simulink model "frequency_synth"  (R2020a)
settings: Solver=VariableStepAuto  StartTime=0.0  StopTime=inf  RelTol=1e-3
undefined symbols (not defined in the file): df
libraries: hdlsllib x36, dsphdlsigops x4
settings Model: Creator=david  LastModifiedBy=david
settings OptimizationCC: BlockReduction=off  ConditionallyExecuteInputs=off  DefaultParameterBehavior=Inlined
settings DebuggingCC: AlgebraicLoopMsg=error
settings HardwareCC: ProdBitPerPointer=32  ProdBitPerSizeT=32  ProdBitPerPtrDiffT=32  ProdLargestAtomicFloat=None  ProdIntDivRoundTo=Undefined  ProdEndianess=Unspecified  ProdWordSize=32  ProdHWDeviceType=ASIC/FPGA->ASIC/FPGA  TargetBitPerPointer=64  TargetBitPerSizeT=64  TargetBitPerPtrDiffT=64  TargetLongLongMode=on  TargetIntDivRoundTo=Zero  TargetEndianess=LittleEndian  TargetWordSize=64  TargetHWDeviceType=Custom Processor->MATLAB Host Computer  ProdEqTarget=off

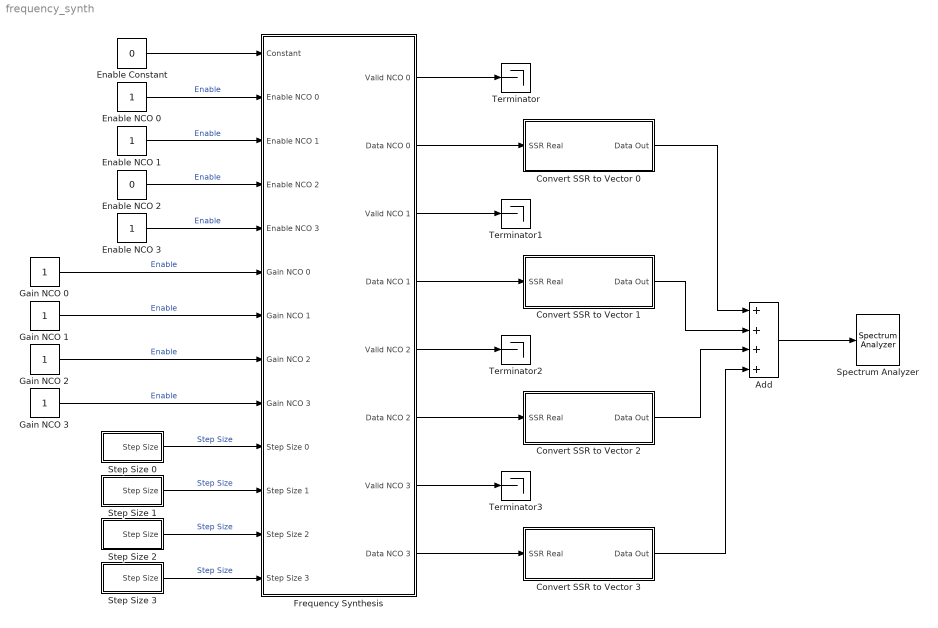
== system frequency_synth ==
  Add : Sum  Inputs=++++
  Convert SSR to Vector 0 : Subsystem
  Convert SSR to Vector 1 : Subsystem
  Convert SSR to Vector 2 : Subsystem
  Convert SSR to Vector 3 : Subsystem
  Enable Constant : Constant  Value=0  OutDataTypeStr=uint32  SampleTime=-1
  Enable NCO 0 : Constant  OutDataTypeStr=boolean  SampleTime=-1
  Enable NCO 1 : Constant  OutDataTypeStr=boolean  SampleTime=-1
  Enable NCO 2 : Constant  Value=0  OutDataTypeStr=boolean  SampleTime=-1
  Enable NCO 3 : Constant  OutDataTypeStr=boolean  SampleTime=-1
  Frequency Synthesis : Subsystem  TreatAsAtomicUnit=on
  Gain NCO {0..3} (4 alike) : Constant  OutDataTypeStr=fixdt(1,16,14)  SampleTime=-1
  Spectrum Analyzer : SpectrumAnalyzer
  Step Size 0 : Subsystem  mask{fs=1.024e9, f=20.1e6, b=32, i=16, ssr=4}
      mask prompts: fs "Sample Frequency (Hz):"; f "Desired Frequency (Hz):"; b "Accumulator Bits:"; i "Quantized Bits:"; ssr "Sample per clock cycle:"
      mask init:
      | N = 2^i;
      | df = (f/fs)*N * 2^(b-i);
  Step Size 1 : Subsystem  mask{fs=1.024e9, f=40.1e6, b=32, i=16, ssr=4}
      mask prompts: fs "Sample Frequency (Hz):"; f "Desired Frequency (Hz):"; b "Accumulator Bits:"; i "Quantized Bits:"; ssr "Sample per clock cycle:"
      mask init:
      | N = 2^i;
      | df = (f/fs)*N * 2^(b-i);
  Step Size 2 : Subsystem  mask{fs=1.024e9, f=80.1e6, b=32, i=16, ssr=4}
      mask prompts: fs "Sample Frequency (Hz):"; f "Desired Frequency (Hz):"; b "Accumulator Bits:"; i "Quantized Bits:"; ssr "Sample per clock cycle:"
      mask init:
      | N = 2^i;
      | df = (f/fs)*N * 2^(b-i);
  Step Size 3 : Subsystem  mask{fs=1.024e9, f=450.01e6, b=32, i=16, ssr=4}
      mask prompts: fs "Sample Frequency (Hz):"; f "Desired Frequency (Hz):"; b "Accumulator Bits:"; i "Quantized Bits:"; ssr "Sample per clock cycle:"
      mask init:
      | N = 2^i;
      | df = (f/fs)*N * 2^(b-i);
  Terminator{,1..3} (4 alike) : Terminator
  wires:
  Step Size 0/1(Step Size) -> Frequency Synthesis/10(Step Size 0)  "Step Size"
  Enable NCO 0/1 -> Frequency Synthesis/2(Enable NCO 0)  "Enable"
  Step Size 1/1(Step Size) -> Frequency Synthesis/11(Step Size 1)  "Step Size"
  Frequency Synthesis/2(Data NCO 0) -> Convert SSR to Vector 0/1(SSR Real)
  Step Size 2/1(Step Size) -> Frequency Synthesis/12(Step Size 2)  "Step Size"
  Step Size 3/1(Step Size) -> Frequency Synthesis/13(Step Size 3)  "Step Size"
  Enable NCO 1/1 -> Frequency Synthesis/3(Enable NCO 1)  "Enable"
  Enable NCO 2/1 -> Frequency Synthesis/4(Enable NCO 2)  "Enable"
  Enable NCO 3/1 -> Frequency Synthesis/5(Enable NCO 3)  "Enable"
  Gain NCO 3/1 -> Frequency Synthesis/9(Gain NCO 3)  "Enable"
  Gain NCO 0/1 -> Frequency Synthesis/6(Gain NCO 0)  "Enable"
  Gain NCO 1/1 -> Frequency Synthesis/7(Gain NCO 1)  "Enable"
  Gain NCO 2/1 -> Frequency Synthesis/8(Gain NCO 2)  "Enable"
  Frequency Synthesis/1(Valid NCO 0) -> Terminator/1
  Frequency Synthesis/3(Valid NCO 1) -> Terminator1/1
  Frequency Synthesis/5(Valid NCO 2) -> Terminator2/1
  Frequency Synthesis/7(Valid NCO 3) -> Terminator3/1
  Add/1 -> Spectrum Analyzer/1
  Convert SSR to Vector 0/1(Data Out) -> Add/1
  Frequency Synthesis/4(Data NCO 1) -> Convert SSR to Vector 1/1(SSR Real)
  Convert SSR to Vector 1/1(Data Out) -> Add/2
  Frequency Synthesis/6(Data NCO 2) -> Convert SSR to Vector 2/1(SSR Real)
  Convert SSR to Vector 2/1(Data Out) -> Add/3
  Frequency Synthesis/8(Data NCO 3) -> Convert SSR to Vector 3/1(SSR Real)
  Convert SSR to Vector 3/1(Data Out) -> Add/4
  Enable Constant/1 -> Frequency Synthesis/1(Constant)

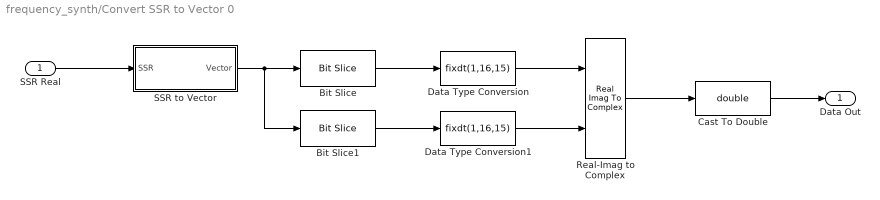
== system frequency_synth/Convert SSR to Vector 0 ==
  SSR Real : Inport
  Bit Slice : hdlsllib/Logic and Bit Operations/Bit Slice  lidx=15  ridx=0
      settings: SourceProductBaseCode=SL
  Bit Slice1 : hdlsllib/Logic and Bit Operations/Bit Slice  lidx=31  ridx=16
      settings: SourceProductBaseCode=SL
  Cast To Double : DataTypeConversion  OutDataTypeStr=double
  Data Type Conversion : DataTypeConversion  OutDataTypeStr=fixdt(1,16,15)  ConvertRealWorld=Stored Integer (SI)
  Data Type Conversion1 : DataTypeConversion  OutDataTypeStr=fixdt(1,16,15)  ConvertRealWorld=Stored Integer (SI)
  Real-Imag to Complex : RealImagToComplex
  SSR to Vector : Subsystem  mask{N=4, w=32, hN=4, hw=32}
      mask prompts: N "Samples per clock cycle:"; w "Wordlength:"
      mask init:
      | if ~isequal(get_param(gcb, 'N'), get_param(gcb, 'hN')) ||...
      |         ~isequal(get_param(gcb, 'w'), get_param(gcb, 'hw'))
      |     % Delete all blocks except input and output ports
      |     delete_block(setxor(setdiff(...
      |         find_system(gcb,'LookUnderMasks','on'),...
      |         {[gcb, '/Vector'], [gcb, '/SSR']}), gcb));
      | 
      |     % Delete all wires
      |     delete_line(find_system(gcb, 'FindAll', 'on', 'LookUnderMasks',...
      |         'on', 'SearchDepth', 3, 'Type', 'line', 'Connected', 'off'));
      | 
      |     % Add the matrix concatenation block
      |     add_block('hdlsllib/Math Operations/Matrix Concatenate',...
      |         [gcb, '/Matrix Concatenate'],...
      |         'Position', [155 55 205 330]);
      |     set_param([gcb, '/Matrix Concatenate'], 'NumInputs', num2str(N));
      |     set_param([gcb, '/Matrix Concatenate'], 'Mode', 'Vector');
      |     
      |     % Add wire to output
      |     add_line(gcb, 'Matrix Concatenate/1', 'Vector/1');
      | 
      |     % Add slice blocks and connect wires
      |     for i = 0:N-1
      |         add_block('hdlsllib/Logic and Bit Operations/Bit Slice',...
      |             [gcb, '/Bit Slice', num2str(i)],...
      |             'Position', [0 82+i*90 45 128+i*90]);
      |         set_param([gcb, '/Bit Slice', num2str(i)], 'ridx', num2str(0+i*(w)));
      |         set_param([gcb, '/Bit Slice', num2str(i)], 'lidx', num2str((w-1)+i*(w)));
      |         add_line(gcb, 'SSR/1', ['Bit Slice', num2str(i), '/1'],...
      |             'autorouting', 'on');
      |         add_line(gcb, ['Bit Slice', num2str(i), '/1'],...
      |             ['Matrix Concatenate/', num2str(i+1)],...
      |             'autorouting', 'on');
      |     end
      |     
      |     % Set the hidden attribute to prevent unnecessary changes in
      |     % architecture while generating HDL Code.
      |     set_param(gcb, 'hN', get_param(gcb, 'N'));
      |     set_param(gcb, 'hw', get_param(gcb, 'w'));
      | end
      mask DialogControl DescGroupVar Prompt: SSR to Vector
      mask DialogControl DescTextVar Prompt: Convert the SSR vector format based on the wordlength and expected number of samples per clock cycle.
  Data Out : Outport
  wires:
  Real-Imag to Complex/1 -> Cast To Double/1
  Data Type Conversion/1 -> Real-Imag to Complex/1
  SSR to Vector/1(Vector) -> Bit Slice1/1, Bit Slice/1
  Data Type Conversion1/1 -> Real-Imag to Complex/2
  SSR Real/1 -> SSR to Vector/1(SSR)
  Bit Slice/1 -> Data Type Conversion/1
  Bit Slice1/1 -> Data Type Conversion1/1
  Cast To Double/1 -> Data Out/1

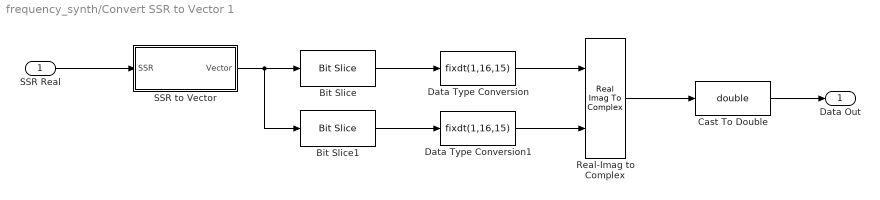
== system frequency_synth/Convert SSR to Vector 1 ==
  SSR Real : Inport
  Bit Slice : hdlsllib/Logic and Bit Operations/Bit Slice  lidx=15  ridx=0
      settings: SourceProductBaseCode=SL
  Bit Slice1 : hdlsllib/Logic and Bit Operations/Bit Slice  lidx=31  ridx=16
      settings: SourceProductBaseCode=SL
  Cast To Double : DataTypeConversion  OutDataTypeStr=double
  Data Type Conversion : DataTypeConversion  OutDataTypeStr=fixdt(1,16,15)  ConvertRealWorld=Stored Integer (SI)
  Data Type Conversion1 : DataTypeConversion  OutDataTypeStr=fixdt(1,16,15)  ConvertRealWorld=Stored Integer (SI)
  Real-Imag to Complex : RealImagToComplex
  SSR to Vector : Subsystem  mask{N=4, w=32, hN=4, hw=32}
      mask prompts: N "Samples per clock cycle:"; w "Wordlength:"
      mask init: same as frequency_synth/Convert SSR to Vector 0/SSR to Vector
      mask DialogControl DescGroupVar Prompt: SSR to Vector
      mask DialogControl DescTextVar Prompt: Convert the SSR vector format based on the wordlength and expected number of samples per clock cycle.
  Data Out : Outport
  wires:
  Cast To Double/1 -> Data Out/1
  Bit Slice1/1 -> Data Type Conversion1/1
  Bit Slice/1 -> Data Type Conversion/1
  SSR Real/1 -> SSR to Vector/1(SSR)
  Data Type Conversion1/1 -> Real-Imag to Complex/2
  SSR to Vector/1(Vector) -> Bit Slice/1, Bit Slice1/1
  Data Type Conversion/1 -> Real-Imag to Complex/1
  Real-Imag to Complex/1 -> Cast To Double/1

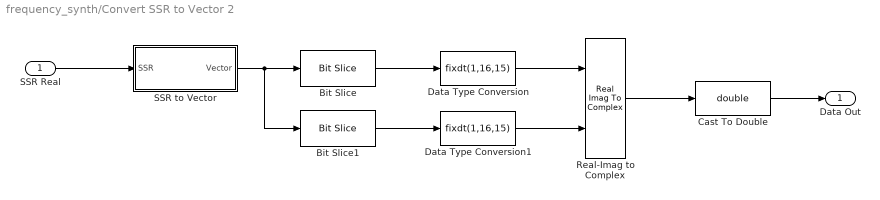
== system frequency_synth/Convert SSR to Vector 2 ==
  SSR Real : Inport
  Bit Slice : hdlsllib/Logic and Bit Operations/Bit Slice  lidx=15  ridx=0
      settings: SourceProductBaseCode=SL
  Bit Slice1 : hdlsllib/Logic and Bit Operations/Bit Slice  lidx=31  ridx=16
      settings: SourceProductBaseCode=SL
  Cast To Double : DataTypeConversion  OutDataTypeStr=double
  Data Type Conversion : DataTypeConversion  OutDataTypeStr=fixdt(1,16,15)  ConvertRealWorld=Stored Integer (SI)
  Data Type Conversion1 : DataTypeConversion  OutDataTypeStr=fixdt(1,16,15)  ConvertRealWorld=Stored Integer (SI)
  Real-Imag to Complex : RealImagToComplex
  SSR to Vector : Subsystem  mask{N=4, w=32, hN=4, hw=32}
      mask prompts: N "Samples per clock cycle:"; w "Wordlength:"
      mask init: same as frequency_synth/Convert SSR to Vector 0/SSR to Vector
      mask DialogControl DescGroupVar Prompt: SSR to Vector
      mask DialogControl DescTextVar Prompt: Convert the SSR vector format based on the wordlength and expected number of samples per clock cycle.
  Data Out : Outport
  wires:
  Real-Imag to Complex/1 -> Cast To Double/1
  Data Type Conversion/1 -> Real-Imag to Complex/1
  SSR to Vector/1(Vector) -> Bit Slice1/1, Bit Slice/1
  Data Type Conversion1/1 -> Real-Imag to Complex/2
  SSR Real/1 -> SSR to Vector/1(SSR)
  Bit Slice/1 -> Data Type Conversion/1
  Bit Slice1/1 -> Data Type Conversion1/1
  Cast To Double/1 -> Data Out/1

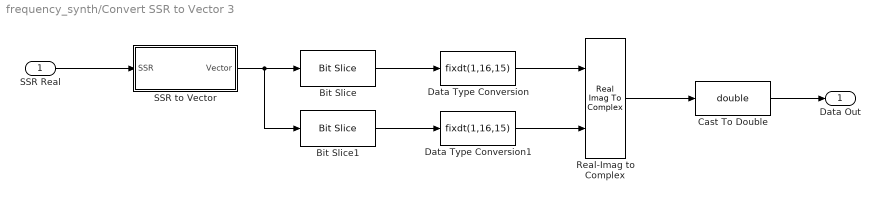
== system frequency_synth/Convert SSR to Vector 3 ==
  SSR Real : Inport
  Bit Slice : hdlsllib/Logic and Bit Operations/Bit Slice  lidx=15  ridx=0
      settings: SourceProductBaseCode=SL
  Bit Slice1 : hdlsllib/Logic and Bit Operations/Bit Slice  lidx=31  ridx=16
      settings: SourceProductBaseCode=SL
  Cast To Double : DataTypeConversion  OutDataTypeStr=double
  Data Type Conversion : DataTypeConversion  OutDataTypeStr=fixdt(1,16,15)  ConvertRealWorld=Stored Integer (SI)
  Data Type Conversion1 : DataTypeConversion  OutDataTypeStr=fixdt(1,16,15)  ConvertRealWorld=Stored Integer (SI)
  Real-Imag to Complex : RealImagToComplex
  SSR to Vector : Subsystem  mask{N=4, w=32, hN=4, hw=32}
      mask prompts: N "Samples per clock cycle:"; w "Wordlength:"
      mask init: same as frequency_synth/Convert SSR to Vector 0/SSR to Vector
      mask DialogControl DescGroupVar Prompt: SSR to Vector
      mask DialogControl DescTextVar Prompt: Convert the SSR vector format based on the wordlength and expected number of samples per clock cycle.
  Data Out : Outport
  wires:
  Cast To Double/1 -> Data Out/1
  Bit Slice1/1 -> Data Type Conversion1/1
  Bit Slice/1 -> Data Type Conversion/1
  SSR Real/1 -> SSR to Vector/1(SSR)
  Data Type Conversion1/1 -> Real-Imag to Complex/2
  SSR to Vector/1(Vector) -> Bit Slice/1, Bit Slice1/1
  Data Type Conversion/1 -> Real-Imag to Complex/1
  Real-Imag to Complex/1 -> Cast To Double/1

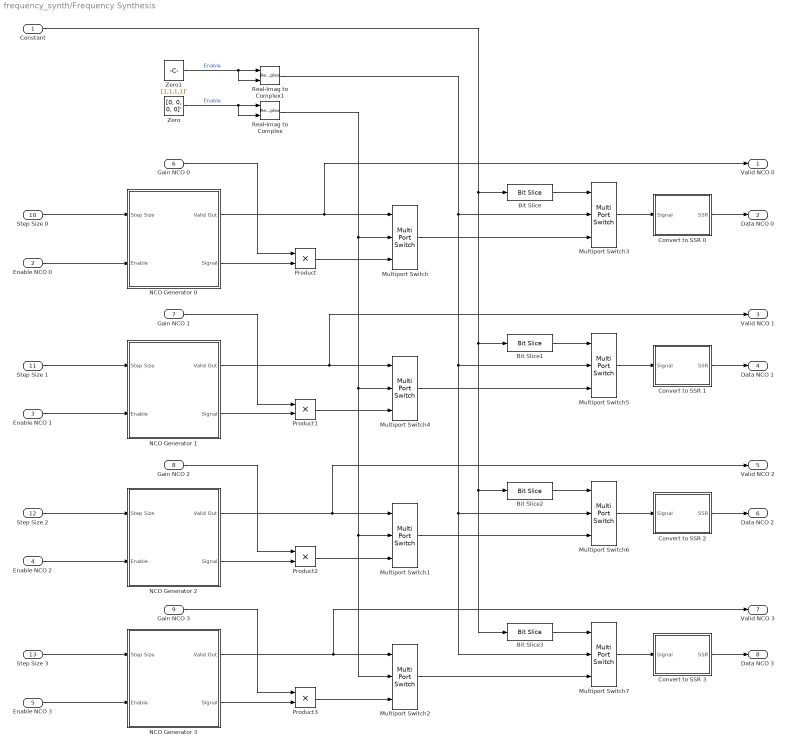
== system frequency_synth/Frequency Synthesis ==
  Constant : Inport
  Enable NCO 0 : Inport  Port=2
  Enable NCO 1 : Inport  Port=3
  Enable NCO 2 : Inport  Port=4
  Enable NCO 3 : Inport  Port=5
  Gain NCO 0 : Inport  Port=6
  Gain NCO 1 : Inport  Port=7
  Gain NCO 2 : Inport  Port=8
  Gain NCO 3 : Inport  Port=9
  Step Size 0 : Inport  Port=10
  Step Size 1 : Inport  Port=11
  Step Size 2 : Inport  Port=12
  Step Size 3 : Inport  Port=13
  Bit Slice : hdlsllib/Logic and Bit Operations/Bit Slice  lidx=0  ridx=0
      settings: SourceProductBaseCode=SL
  Bit Slice1 : hdlsllib/Logic and Bit Operations/Bit Slice  lidx=1  ridx=1
      settings: SourceProductBaseCode=SL
  Bit Slice2 : hdlsllib/Logic and Bit Operations/Bit Slice  lidx=2  ridx=2
      settings: SourceProductBaseCode=SL
  Bit Slice3 : hdlsllib/Logic and Bit Operations/Bit Slice  lidx=3  ridx=3
      settings: SourceProductBaseCode=SL
  Convert to SSR 0 : Subsystem
  Convert to SSR 1 : Subsystem
  Convert to SSR 2 : Subsystem
  Convert to SSR 3 : Subsystem
  Multiport Switch{,1..7} (8 alike) : MultiPortSwitch  DataPortOrder=Zero-based contiguous  Inputs=2  zeroidx=on
  NCO Generator 0 : Subsystem  mask{fs=1.024e9, b=32, i=16, ssr=4}
      mask prompts: fs "Sample Frequency (Hz):"; b "Accumulator Bits:"; i "Quantized Bits:"; ssr "Samples per clock cycle:"
  NCO Generator 1 : Subsystem  mask{fs=1.024e9, b=32, i=16, ssr=4}
      mask prompts: fs "Sample Frequency (Hz):"; b "Accumulator Bits:"; i "Quantized Bits:"; ssr "Samples per clock cycle:"
  NCO Generator 2 : Subsystem  mask{fs=1.024e9, b=32, i=16, ssr=4}
      mask prompts: fs "Sample Frequency (Hz):"; b "Accumulator Bits:"; i "Quantized Bits:"; ssr "Samples per clock cycle:"
  NCO Generator 3 : Subsystem  mask{fs=1.024e9, b=32, i=16, ssr=4}
      mask prompts: fs "Sample Frequency (Hz):"; b "Accumulator Bits:"; i "Quantized Bits:"; ssr "Samples per clock cycle:"
  Product{,1..3} (4 alike) : Product  OutDataTypeStr=fixdt(1,16,15)
  Real-Imag to Complex : RealImagToComplex
  Real-Imag to Complex1 : RealImagToComplex
  Zero : Constant  Value=[0, 0, 0, 0]'  VectorParams1D=off  OutDataTypeStr=fixdt(1,16,15)  SampleTime=-1
  Zero1 : Constant  Value=[1,1,1,1]'  VectorParams1D=off  OutDataTypeStr=fixdt(1,16,15)  SampleTime=-1
  Valid NCO 0 : Outport
  Data NCO 0 : Outport  Port=2
  Valid NCO 1 : Outport  Port=3
  Data NCO 1 : Outport  Port=4
  Valid NCO 2 : Outport  Port=5
  Data NCO 2 : Outport  Port=6
  Valid NCO 3 : Outport  Port=7
  Data NCO 3 : Outport  Port=8
  wires:
  Step Size 0/1 -> NCO Generator 0/1(Step Size)
  Step Size 1/1 -> NCO Generator 1/1(Step Size)
  Enable NCO 0/1 -> NCO Generator 0/2(Enable)
  Step Size 2/1 -> NCO Generator 2/1(Step Size)
  Step Size 3/1 -> NCO Generator 3/1(Step Size)
  NCO Generator 0/2(Signal) -> Product/2
  Enable NCO 1/1 -> NCO Generator 1/2(Enable)
  Enable NCO 2/1 -> NCO Generator 2/2(Enable)
  Enable NCO 3/1 -> NCO Generator 3/2(Enable)
  Gain NCO 0/1 -> Product/1
  NCO Generator 1/2(Signal) -> Product1/2
  Gain NCO 1/1 -> Product1/1
  NCO Generator 2/2(Signal) -> Product2/2
  Gain NCO 2/1 -> Product2/1
  NCO Generator 3/2(Signal) -> Product3/2
  Gain NCO 3/1 -> Product3/1
  Product/1 -> Multiport Switch/3
  NCO Generator 0/1(Valid Out) -> Valid NCO 0/1, Multiport Switch/1
  Product1/1 -> Multiport Switch4/3
  NCO Generator 1/1(Valid Out) -> Valid NCO 1/1, Multiport Switch4/1
  Product2/1 -> Multiport Switch1/3
  NCO Generator 2/1(Valid Out) -> Valid NCO 2/1, Multiport Switch1/1
  Product3/1 -> Multiport Switch2/3
  NCO Generator 3/1(Valid Out) -> Valid NCO 3/1, Multiport Switch2/1
  Zero/1 -> Real-Imag to Complex/2, Real-Imag to Complex/1  "Enable"
  Real-Imag to Complex/1 -> Multiport Switch2/2, Multiport Switch1/2, Multiport Switch4/2, Multiport Switch/2
  Convert to SSR 0/1(SSR) -> Data NCO 0/1
  Convert to SSR 1/1(SSR) -> Data NCO 1/1
  Convert to SSR 2/1(SSR) -> Data NCO 2/1
  Convert to SSR 3/1(SSR) -> Data NCO 3/1
  Zero1/1 -> Real-Imag to Complex1/2, Real-Imag to Complex1/1  "Enable"
  Multiport Switch/1 -> Multiport Switch3/3
  Multiport Switch3/1 -> Convert to SSR 0/1(Signal)
  Real-Imag to Complex1/1 -> Multiport Switch3/2, Multiport Switch5/2, Multiport Switch6/2, Multiport Switch7/2
  Constant/1 -> Bit Slice1/1, Bit Slice2/1, Bit Slice3/1, Bit Slice/1
  Multiport Switch4/1 -> Multiport Switch5/3
  Multiport Switch5/1 -> Convert to SSR 1/1(Signal)
  Multiport Switch1/1 -> Multiport Switch6/3
  Multiport Switch6/1 -> Convert to SSR 2/1(Signal)
  Multiport Switch2/1 -> Multiport Switch7/3
  Multiport Switch7/1 -> Convert to SSR 3/1(Signal)
  Bit Slice/1 -> Multiport Switch3/1
  Bit Slice1/1 -> Multiport Switch5/1
  Bit Slice2/1 -> Multiport Switch6/1
  Bit Slice3/1 -> Multiport Switch7/1

== system frequency_synth/Step Size 0 ==
  Constant1 : Constant  Value=df  OutDataTypeStr=fixdt(0,b,0)  SampleTime=1/(fs/ssr)
  Step Size : Outport
  wires:
  Constant1/1 -> Step Size/1

== system frequency_synth/Step Size 1 ==
  Constant1 : Constant  Value=df  OutDataTypeStr=fixdt(0,b,0)  SampleTime=1/(fs/ssr)
  Step Size : Outport
  wires:
  Constant1/1 -> Step Size/1

== system frequency_synth/Step Size 2 ==
  Constant1 : Constant  Value=df  OutDataTypeStr=fixdt(0,b,0)  SampleTime=1/(fs/ssr)
  Step Size : Outport
  wires:
  Constant1/1 -> Step Size/1

== system frequency_synth/Step Size 3 ==
  Constant1 : Constant  Value=df  OutDataTypeStr=fixdt(0,b,0)  SampleTime=1/(fs/ssr)
  Step Size : Outport
  wires:
  Constant1/1 -> Step Size/1

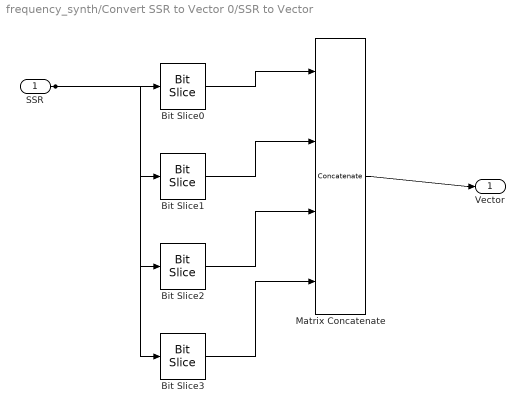
== system frequency_synth/Convert SSR to Vector 0/SSR to Vector ==
  SSR : Inport
  Bit Slice0 : hdlsllib/Logic and Bit Operations/Bit Slice  lidx=31  ridx=0
      settings: SourceProductBaseCode=SL
  Bit Slice1 : hdlsllib/Logic and Bit Operations/Bit Slice  lidx=63  ridx=32
      settings: SourceProductBaseCode=SL
  Bit Slice2 : hdlsllib/Logic and Bit Operations/Bit Slice  lidx=95  ridx=64
      settings: SourceProductBaseCode=SL
  Bit Slice3 : hdlsllib/Logic and Bit Operations/Bit Slice  lidx=127  ridx=96
      settings: SourceProductBaseCode=SL
  Matrix Concatenate : Concatenate  NumInputs=4  ConcatenateDimension=2
  Vector : Outport
  wires:
  Matrix Concatenate/1 -> Vector/1
  SSR/1 -> Bit Slice0/1, Bit Slice1/1, Bit Slice2/1, Bit Slice3/1
  Bit Slice0/1 -> Matrix Concatenate/1
  Bit Slice1/1 -> Matrix Concatenate/2
  Bit Slice2/1 -> Matrix Concatenate/3
  Bit Slice3/1 -> Matrix Concatenate/4

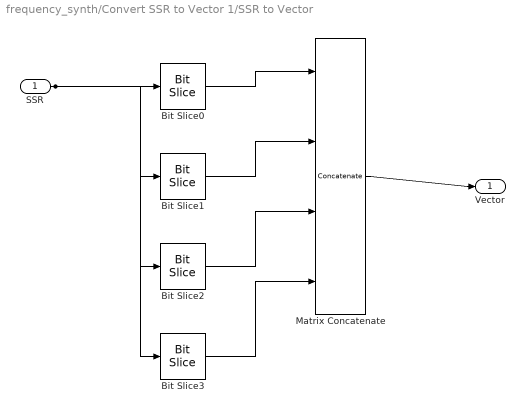
== system frequency_synth/Convert SSR to Vector 1/SSR to Vector ==
  SSR : Inport
  Bit Slice0 : hdlsllib/Logic and Bit Operations/Bit Slice  lidx=31  ridx=0
      settings: SourceProductBaseCode=SL
  Bit Slice1 : hdlsllib/Logic and Bit Operations/Bit Slice  lidx=63  ridx=32
      settings: SourceProductBaseCode=SL
  Bit Slice2 : hdlsllib/Logic and Bit Operations/Bit Slice  lidx=95  ridx=64
      settings: SourceProductBaseCode=SL
  Bit Slice3 : hdlsllib/Logic and Bit Operations/Bit Slice  lidx=127  ridx=96
      settings: SourceProductBaseCode=SL
  Matrix Concatenate : Concatenate  NumInputs=4  ConcatenateDimension=2
  Vector : Outport
  wires:
  Bit Slice3/1 -> Matrix Concatenate/4
  Bit Slice2/1 -> Matrix Concatenate/3
  Bit Slice1/1 -> Matrix Concatenate/2
  Bit Slice0/1 -> Matrix Concatenate/1
  SSR/1 -> Bit Slice3/1, Bit Slice2/1, Bit Slice1/1, Bit Slice0/1
  Matrix Concatenate/1 -> Vector/1

== system frequency_synth/Convert SSR to Vector 2/SSR to Vector ==
  SSR : Inport
  Bit Slice0 : hdlsllib/Logic and Bit Operations/Bit Slice  lidx=31  ridx=0
      settings: SourceProductBaseCode=SL
  Bit Slice1 : hdlsllib/Logic and Bit Operations/Bit Slice  lidx=63  ridx=32
      settings: SourceProductBaseCode=SL
  Bit Slice2 : hdlsllib/Logic and Bit Operations/Bit Slice  lidx=95  ridx=64
      settings: SourceProductBaseCode=SL
  Bit Slice3 : hdlsllib/Logic and Bit Operations/Bit Slice  lidx=127  ridx=96
      settings: SourceProductBaseCode=SL
  Matrix Concatenate : Concatenate  NumInputs=4  ConcatenateDimension=2
  Vector : Outport
  wires:
  Matrix Concatenate/1 -> Vector/1
  SSR/1 -> Bit Slice0/1, Bit Slice1/1, Bit Slice2/1, Bit Slice3/1
  Bit Slice0/1 -> Matrix Concatenate/1
  Bit Slice1/1 -> Matrix Concatenate/2
  Bit Slice2/1 -> Matrix Concatenate/3
  Bit Slice3/1 -> Matrix Concatenate/4

== system frequency_synth/Convert SSR to Vector 3/SSR to Vector ==
  SSR : Inport
  Bit Slice0 : hdlsllib/Logic and Bit Operations/Bit Slice  lidx=31  ridx=0
      settings: SourceProductBaseCode=SL
  Bit Slice1 : hdlsllib/Logic and Bit Operations/Bit Slice  lidx=63  ridx=32
      settings: SourceProductBaseCode=SL
  Bit Slice2 : hdlsllib/Logic and Bit Operations/Bit Slice  lidx=95  ridx=64
      settings: SourceProductBaseCode=SL
  Bit Slice3 : hdlsllib/Logic and Bit Operations/Bit Slice  lidx=127  ridx=96
      settings: SourceProductBaseCode=SL
  Matrix Concatenate : Concatenate  NumInputs=4  ConcatenateDimension=2
  Vector : Outport
  wires:
  Bit Slice3/1 -> Matrix Concatenate/4
  Bit Slice2/1 -> Matrix Concatenate/3
  Bit Slice1/1 -> Matrix Concatenate/2
  Bit Slice0/1 -> Matrix Concatenate/1
  SSR/1 -> Bit Slice3/1, Bit Slice2/1, Bit Slice1/1, Bit Slice0/1
  Matrix Concatenate/1 -> Vector/1

== system frequency_synth/Frequency Synthesis/Convert to SSR 0 ==
  Signal : Inport
  Bit Concat : hdlsllib/Logic and Bit Operations/Bit Concat  numInputs=2
  Complex to Real-Imag : ComplexToRealImag
  Vector to SSR Low : Subsystem  mask{N=4, hN=4}
      mask prompts: N "Samples per clock cycle:"
      mask init:
      | if ~isequal(get_param(gcb, 'N'), get_param(gcb, 'hN'))
      |     % Delete all blocks except input and output ports
      |     delete_block(setxor(setdiff(...
      |         find_system(gcb,'LookUnderMasks','on'),...
      |         {[gcb, '/Vector'], [gcb, '/SSR']}), gcb));
      | 
      |     % Delete all wires
      |     delete_line(find_system(gcb, 'FindAll', 'on', 'LookUnderMasks',...
      |         'on', 'SearchDepth', 3, 'Type', 'line', 'Connected', 'off'));
      | 
      |     % Add the bit concatenation block
      |     add_block('hdlsllib/Logic and Bit Operations/Bit Concat',...
      |         [gcb, '/Bit Concat'],...
      |         'Position', [155 55 205 330]);
      |     set_param([gcb, '/Bit Concat'], 'numInputs', num2str(N));
      | 
      |     % Add wire to output
      |     add_line(gcb, 'Bit Concat/1', 'SSR/1');
      | 
      |     % Add selector blocks and connect wires
      |     for i = 0:N-1
      |         add_block('simulink/Signal Routing/Selector',...
      |             [gcb, '/Selector', num2str(i)],...
      |             'Position', [0 82+i*90 45 128+i*90]);
      |         set_param([gcb, '/Selector', num2str(i)], 'InputPortWidth', num2str(N));
      |         set_param([gcb, '/Selector', num2str(i)], 'IndexParamArray', {num2str(N-i)});
      |         add_line(gcb, 'Vector/1', ['Selector', num2str(i), '/1'],...
      |             'autorouting', 'on');
      |         add_line(gcb, ['Selector', num2str(i), '/1'],...
      |             ['Bit Concat/', num2str(i+1)],...
      |             'autorouting', 'on');
      |     end
      |     
      |     % Set the hidden attribute to prevent unnecessary changes in
      |     % architecture while generating HDL Code.
      |     set_param(gcb, 'hN', get_param(gcb, 'N'));
      | end
      mask DialogControl DescGroupVar Prompt: Vector to SSR
      mask DialogControl DescTextVar Prompt: Convert a vector of inputs into SSR format.
  SSR : Outport
  wires:
  Bit Concat/1 -> Vector to SSR Low/1(Vector)
  Complex to Real-Imag/2 -> Bit Concat/1
  Complex to Real-Imag/1 -> Bit Concat/2
  Vector to SSR Low/1(SSR) -> SSR/1
  Signal/1 -> Complex to Real-Imag/1

== system frequency_synth/Frequency Synthesis/Convert to SSR 1 ==
  Signal : Inport
  Bit Concat : hdlsllib/Logic and Bit Operations/Bit Concat  numInputs=2
  Complex to Real-Imag : ComplexToRealImag
  Vector to SSR Low : Subsystem  mask{N=4, hN=4}
      mask prompts: N "Samples per clock cycle:"
      mask init: same as frequency_synth/Frequency Synthesis/Convert to SSR 0/Vector to SSR Low
      mask DialogControl DescGroupVar Prompt: Vector to SSR
      mask DialogControl DescTextVar Prompt: Convert a vector of inputs into SSR format.
  SSR : Outport
  wires:
  Signal/1 -> Complex to Real-Imag/1
  Vector to SSR Low/1(SSR) -> SSR/1
  Complex to Real-Imag/1 -> Bit Concat/2
  Complex to Real-Imag/2 -> Bit Concat/1
  Bit Concat/1 -> Vector to SSR Low/1(Vector)

== system frequency_synth/Frequency Synthesis/Convert to SSR 2 ==
  Signal : Inport
  Bit Concat : hdlsllib/Logic and Bit Operations/Bit Concat  numInputs=2
  Complex to Real-Imag : ComplexToRealImag
  Vector to SSR Low : Subsystem  mask{N=4, hN=4}
      mask prompts: N "Samples per clock cycle:"
      mask init: same as frequency_synth/Frequency Synthesis/Convert to SSR 0/Vector to SSR Low
      mask DialogControl DescGroupVar Prompt: Vector to SSR
      mask DialogControl DescTextVar Prompt: Convert a vector of inputs into SSR format.
  SSR : Outport
  wires:
  Bit Concat/1 -> Vector to SSR Low/1(Vector)
  Complex to Real-Imag/2 -> Bit Concat/1
  Complex to Real-Imag/1 -> Bit Concat/2
  Vector to SSR Low/1(SSR) -> SSR/1
  Signal/1 -> Complex to Real-Imag/1

== system frequency_synth/Frequency Synthesis/Convert to SSR 3 ==
  Signal : Inport
  Bit Concat : hdlsllib/Logic and Bit Operations/Bit Concat  numInputs=2
  Complex to Real-Imag : ComplexToRealImag
  Vector to SSR Low : Subsystem  mask{N=4, hN=4}
      mask prompts: N "Samples per clock cycle:"
      mask init: same as frequency_synth/Frequency Synthesis/Convert to SSR 0/Vector to SSR Low
      mask DialogControl DescGroupVar Prompt: Vector to SSR
      mask DialogControl DescTextVar Prompt: Convert a vector of inputs into SSR format.
  SSR : Outport
  wires:
  Signal/1 -> Complex to Real-Imag/1
  Vector to SSR Low/1(SSR) -> SSR/1
  Complex to Real-Imag/1 -> Bit Concat/2
  Complex to Real-Imag/2 -> Bit Concat/1
  Bit Concat/1 -> Vector to SSR Low/1(Vector)

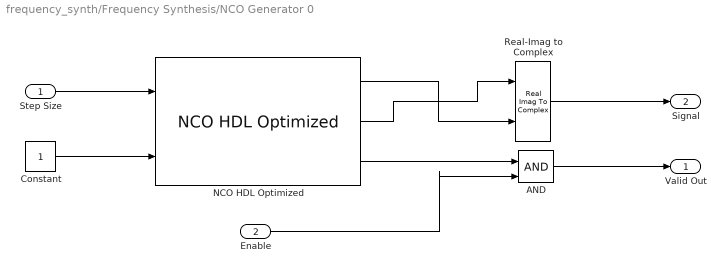
== system frequency_synth/Frequency Synthesis/NCO Generator 0 ==
  Step Size : Inport
  Enable : Inport  Port=2
  AND : Logic  IconShape=distinctive  AllPortsSameDT=off  OutDataTypeStr=boolean
  Constant : Constant  OutDataTypeStr=boolean  SampleTime=1/(fs/ssr)
  NCO HDL Optimized : dsphdlsigops/NCO HDL Optimized  PhaseIncrementSource=Input port  PhaseIncrement=fix(df)  PhaseOffsetSource=Property  PhaseOffset=0  DitherSource=None  NumDitherBits=8  SamplesPerFrame=ssr  LUTCompress=on  ResetAction=off  Waveform=Sine and cosine  PhasePort=off  SimulateUsing=Code generation  AccumulatorWL=b  PhaseQuantization=on  NumQuantizerAccumulatorBits=i  OutputDataType=Binary point scaling  OutputWL=16  OutputFL=15
      settings: SourceProductBaseCode=DS
  Real-Imag to Complex : RealImagToComplex
  Valid Out : Outport
  Signal : Outport  Port=2
  wires:
  Real-Imag to Complex/1 -> Signal/1
  NCO HDL Optimized/1 -> Real-Imag to Complex/2
  NCO HDL Optimized/2 -> Real-Imag to Complex/1
  Step Size/1 -> NCO HDL Optimized/1
  Constant/1 -> NCO HDL Optimized/2
  Enable/1 -> AND/2
  NCO HDL Optimized/3 -> AND/1
  AND/1 -> Valid Out/1

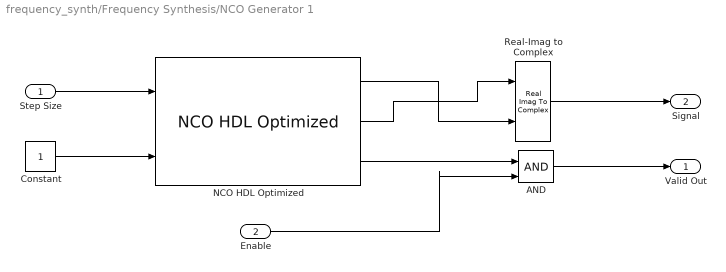
== system frequency_synth/Frequency Synthesis/NCO Generator 1 ==
  Step Size : Inport
  Enable : Inport  Port=2
  AND : Logic  IconShape=distinctive  AllPortsSameDT=off  OutDataTypeStr=boolean
  Constant : Constant  OutDataTypeStr=boolean  SampleTime=1/(fs/ssr)
  NCO HDL Optimized : dsphdlsigops/NCO HDL Optimized  PhaseIncrementSource=Input port  PhaseIncrement=fix(df)  PhaseOffsetSource=Property  PhaseOffset=0  DitherSource=None  NumDitherBits=8  SamplesPerFrame=ssr  LUTCompress=on  ResetAction=off  Waveform=Sine and cosine  PhasePort=off  SimulateUsing=Code generation  AccumulatorWL=b  PhaseQuantization=on  NumQuantizerAccumulatorBits=i  OutputDataType=Binary point scaling  OutputWL=16  OutputFL=15
      settings: SourceProductBaseCode=DS
  Real-Imag to Complex : RealImagToComplex
  Valid Out : Outport
  Signal : Outport  Port=2
  wires:
  AND/1 -> Valid Out/1
  NCO HDL Optimized/3 -> AND/1
  Enable/1 -> AND/2
  Constant/1 -> NCO HDL Optimized/2
  Step Size/1 -> NCO HDL Optimized/1
  NCO HDL Optimized/2 -> Real-Imag to Complex/1
  NCO HDL Optimized/1 -> Real-Imag to Complex/2
  Real-Imag to Complex/1 -> Signal/1

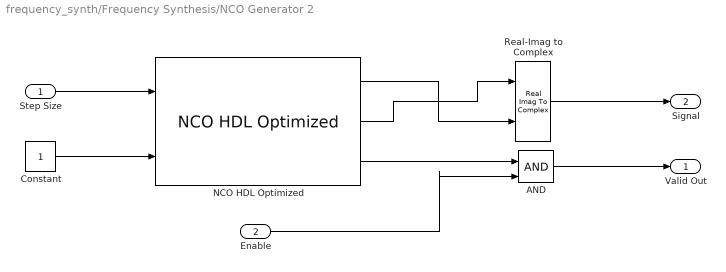
== system frequency_synth/Frequency Synthesis/NCO Generator 2 ==
  Step Size : Inport
  Enable : Inport  Port=2
  AND : Logic  IconShape=distinctive  AllPortsSameDT=off  OutDataTypeStr=boolean
  Constant : Constant  OutDataTypeStr=boolean  SampleTime=1/(fs/ssr)
  NCO HDL Optimized : dsphdlsigops/NCO HDL Optimized  PhaseIncrementSource=Input port  PhaseIncrement=fix(df)  PhaseOffsetSource=Property  PhaseOffset=0  DitherSource=None  NumDitherBits=8  SamplesPerFrame=ssr  LUTCompress=on  ResetAction=off  Waveform=Sine and cosine  PhasePort=off  SimulateUsing=Code generation  AccumulatorWL=b  PhaseQuantization=on  NumQuantizerAccumulatorBits=i  OutputDataType=Binary point scaling  OutputWL=16  OutputFL=15
      settings: SourceProductBaseCode=DS
  Real-Imag to Complex : RealImagToComplex
  Valid Out : Outport
  Signal : Outport  Port=2
  wires:
  Real-Imag to Complex/1 -> Signal/1
  NCO HDL Optimized/1 -> Real-Imag to Complex/2
  NCO HDL Optimized/2 -> Real-Imag to Complex/1
  Step Size/1 -> NCO HDL Optimized/1
  Constant/1 -> NCO HDL Optimized/2
  Enable/1 -> AND/2
  NCO HDL Optimized/3 -> AND/1
  AND/1 -> Valid Out/1

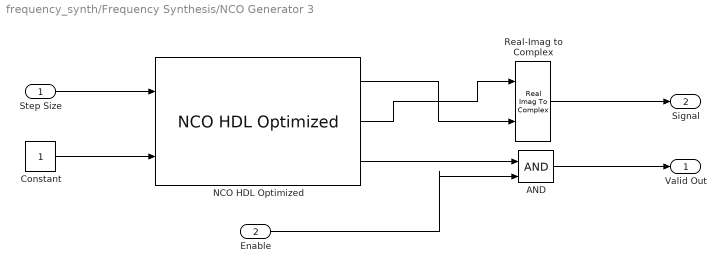
== system frequency_synth/Frequency Synthesis/NCO Generator 3 ==
  Step Size : Inport
  Enable : Inport  Port=2
  AND : Logic  IconShape=distinctive  AllPortsSameDT=off  OutDataTypeStr=boolean
  Constant : Constant  OutDataTypeStr=boolean  SampleTime=1/(fs/ssr)
  NCO HDL Optimized : dsphdlsigops/NCO HDL Optimized  PhaseIncrementSource=Input port  PhaseIncrement=fix(df)  PhaseOffsetSource=Property  PhaseOffset=0  DitherSource=None  NumDitherBits=8  SamplesPerFrame=ssr  LUTCompress=on  ResetAction=off  Waveform=Sine and cosine  PhasePort=off  SimulateUsing=Code generation  AccumulatorWL=b  PhaseQuantization=on  NumQuantizerAccumulatorBits=i  OutputDataType=Binary point scaling  OutputWL=16  OutputFL=15
      settings: SourceProductBaseCode=DS
  Real-Imag to Complex : RealImagToComplex
  Valid Out : Outport
  Signal : Outport  Port=2
  wires:
  AND/1 -> Valid Out/1
  NCO HDL Optimized/3 -> AND/1
  Enable/1 -> AND/2
  Constant/1 -> NCO HDL Optimized/2
  Step Size/1 -> NCO HDL Optimized/1
  NCO HDL Optimized/2 -> Real-Imag to Complex/1
  NCO HDL Optimized/1 -> Real-Imag to Complex/2
  Real-Imag to Complex/1 -> Signal/1

== system frequency_synth/Frequency Synthesis/Convert to SSR 0/Vector to SSR Low ==
  Vector : Inport
  Bit Concat : hdlsllib/Logic and Bit Operations/Bit Concat  numInputs=4
  Selector0 : Selector  InputPortWidth=4  IndexOptions=Index vector (dialog)  Indices=4  OutputSizes=1
  Selector1 : Selector  InputPortWidth=4  IndexOptions=Index vector (dialog)  Indices=3  OutputSizes=1
  Selector2 : Selector  InputPortWidth=4  IndexOptions=Index vector (dialog)  Indices=2  OutputSizes=1
  Selector3 : Selector  InputPortWidth=4  IndexOptions=Index vector (dialog)  Indices=1  OutputSizes=1
  SSR : Outport
  wires:
  Selector3/1 -> Bit Concat/4
  Selector2/1 -> Bit Concat/3
  Selector1/1 -> Bit Concat/2
  Selector0/1 -> Bit Concat/1
  Vector/1 -> Selector3/1, Selector2/1, Selector1/1, Selector0/1
  Bit Concat/1 -> SSR/1

== system frequency_synth/Frequency Synthesis/Convert to SSR 1/Vector to SSR Low ==
  Vector : Inport
  Bit Concat : hdlsllib/Logic and Bit Operations/Bit Concat  numInputs=4
  Selector0 : Selector  InputPortWidth=4  IndexOptions=Index vector (dialog)  Indices=4  OutputSizes=1
  Selector1 : Selector  InputPortWidth=4  IndexOptions=Index vector (dialog)  Indices=3  OutputSizes=1
  Selector2 : Selector  InputPortWidth=4  IndexOptions=Index vector (dialog)  Indices=2  OutputSizes=1
  Selector3 : Selector  InputPortWidth=4  IndexOptions=Index vector (dialog)  Indices=1  OutputSizes=1
  SSR : Outport
  wires:
  Bit Concat/1 -> SSR/1
  Vector/1 -> Selector0/1, Selector1/1, Selector2/1, Selector3/1
  Selector0/1 -> Bit Concat/1
  Selector1/1 -> Bit Concat/2
  Selector2/1 -> Bit Concat/3
  Selector3/1 -> Bit Concat/4

== system frequency_synth/Frequency Synthesis/Convert to SSR 2/Vector to SSR Low ==
  Vector : Inport
  Bit Concat : hdlsllib/Logic and Bit Operations/Bit Concat  numInputs=4
  Selector0 : Selector  InputPortWidth=4  IndexOptions=Index vector (dialog)  Indices=4  OutputSizes=1
  Selector1 : Selector  InputPortWidth=4  IndexOptions=Index vector (dialog)  Indices=3  OutputSizes=1
  Selector2 : Selector  InputPortWidth=4  IndexOptions=Index vector (dialog)  Indices=2  OutputSizes=1
  Selector3 : Selector  InputPortWidth=4  IndexOptions=Index vector (dialog)  Indices=1  OutputSizes=1
  SSR : Outport
  wires:
  Selector3/1 -> Bit Concat/4
  Selector2/1 -> Bit Concat/3
  Selector1/1 -> Bit Concat/2
  Selector0/1 -> Bit Concat/1
  Vector/1 -> Selector3/1, Selector2/1, Selector1/1, Selector0/1
  Bit Concat/1 -> SSR/1

== system frequency_synth/Frequency Synthesis/Convert to SSR 3/Vector to SSR Low ==
  Vector : Inport
  Bit Concat : hdlsllib/Logic and Bit Operations/Bit Concat  numInputs=4
  Selector0 : Selector  InputPortWidth=4  IndexOptions=Index vector (dialog)  Indices=4  OutputSizes=1
  Selector1 : Selector  InputPortWidth=4  IndexOptions=Index vector (dialog)  Indices=3  OutputSizes=1
  Selector2 : Selector  InputPortWidth=4  IndexOptions=Index vector (dialog)  Indices=2  OutputSizes=1
  Selector3 : Selector  InputPortWidth=4  IndexOptions=Index vector (dialog)  Indices=1  OutputSizes=1
  SSR : Outport
  wires:
  Bit Concat/1 -> SSR/1
  Vector/1 -> Selector0/1, Selector1/1, Selector2/1, Selector3/1
  Selector0/1 -> Bit Concat/1
  Selector1/1 -> Bit Concat/2
  Selector2/1 -> Bit Concat/3
  Selector3/1 -> Bit Concat/4
